simulink model "SAS"  (R2018a)
settings: Solver=VariableStepAuto  StartTime=0.0  StopTime=S.simtime  RelTol=1e-3
undefined symbols (not defined in the file): S
libraries: peGeneralControl x1
settings Model: Creator=Can Bekar  LastModifiedBy=Can Bekar
settings DataIOCC: ExternalInput=S.usignal  InitialState=xu  LoadExternalInput=on  SignalLogging=off  DSMLogging=off

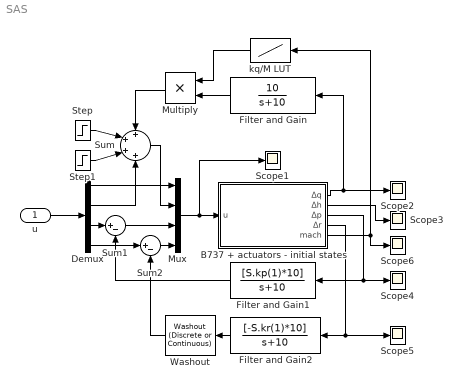
== system SAS ==
  u : Inport
  B737 + actuators - initial states : Subsystem
  Demux : Demux
  Filter and Gain : TransferFcn  Numerator=[10]  Denominator=[1 10]
  Filter and Gain1 : TransferFcn  Numerator=[S.kp(1)*10]  Denominator=[1 10]
  Filter and Gain2 : TransferFcn  Numerator=[-S.kr(1)*10]  Denominator=[1 10]
  Multiply : Product
  Mux : Mux
  Scope{1..6} (6 alike) : Scope
  Step : Step  Time=2  Before=deg2rad(1)  After=deg2rad(-1)  SampleTime=0
  Step1 : Step  After=deg2rad(1)  SampleTime=0
  Sum : Sum  Inputs=++++
  Sum1 : Sum  Inputs=|+-
  Sum2 : Sum  Inputs=|+-
  Washout : peGeneralControl/Washout (Discrete or Continuous)  T=1  Ts=-1
  kq/M LUT : Lookup_n-D  NumberOfTableDimensions=1  BreakpointsForDimension1=[0.2570 0.2590 0.2620 0.2640 0.2660 0.3510 0.3570 0.4200 0.4360 0.4520 0.4690 0.5440 0.5650 0.5870 0.6100 0.6340 0.6590 0.6850 0.7130 0.7270 0.7570 0.7800 0.7801 0.7802 0.7803 0.7804]  Table=S.kqLUT(:,2)  InternalRulePriority=Speed  RndMeth=Simplest  InputSameDT=on
  wires:
  Demux/1 -> Mux/1
  Sum/1 -> Mux/2
  Demux/2 -> Sum/4
  Mux/1 -> Scope1/1, B737 + actuators - initial states/1(u)
  u/1 -> Demux/1
  Step1/1 -> Sum/3
  Step/1 -> Sum/2
  Sum1/1 -> Mux/3
  Demux/3 -> Sum1/1
  Sum2/1 -> Mux/4
  Demux/4 -> Sum2/1
  Filter and Gain1/1 -> Sum1/2
  Filter and Gain2/1 -> Washout/1
  Washout/1 -> Sum2/2
  B737 + actuators - initial states/4(Δr) -> Scope5/1, Filter and Gain2/1
  B737 + actuators - initial states/1(Δq) -> Scope2/1, Filter and Gain/1
  B737 + actuators - initial states/3(Δp) -> Filter and Gain1/1, Scope4/1
  B737 + actuators - initial states/2(Δh) -> Scope3/1
  Filter and Gain/1 -> Multiply/2
  Multiply/1 -> Sum/1
  kq/M LUT/1 -> Multiply/1
  B737 + actuators - initial states/5(mach) -> Scope6/1, kq/M LUT/1

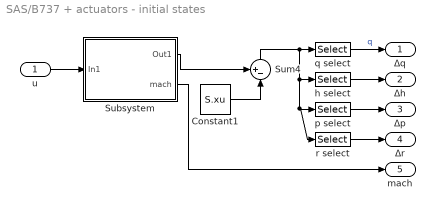
== system SAS/B737 + actuators - initial states ==
  u : Inport
  Constant1 : Constant  Value=S.xu
  Subsystem : Subsystem
  Sum4 : Sum  Inputs=+-|
  h select : Selector  InputPortWidth=12  IndexOptions=Index vector (dialog)  Indices=[12]  OutputSizes=1
  p select : Selector  InputPortWidth=12  IndexOptions=Index vector (dialog)  Indices=[7]  OutputSizes=1
  q select : Selector  InputPortWidth=12  IndexOptions=Index vector (dialog)  Indices=[8]  OutputSizes=1
  r select : Selector  InputPortWidth=12  IndexOptions=Index vector (dialog)  Indices=[9]  OutputSizes=1
  Δq : Outport
  Δh : Outport  Port=2
  Δp : Outport  Port=3
  Δr : Outport  Port=4
  mach : Outport  Port=5
  wires:
  q select/1 -> Δq/1  "q"
  r select/1 -> Δr/1
  Sum4/1 -> r select/1, p select/1, h select/1, q select/1
  Subsystem/1(Out1) -> Sum4/1
  u/1 -> Subsystem/1(In1)
  Constant1/1 -> Sum4/2
  h select/1 -> Δh/1
  p select/1 -> Δp/1
  Subsystem/2(mach) -> mach/1

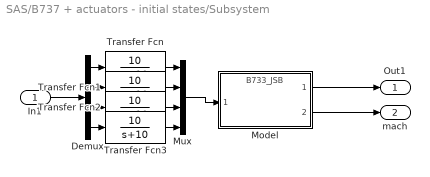
== system SAS/B737 + actuators - initial states/Subsystem ==
  In1 : Inport
  Demux : Demux
  Model : ModelReference  ModelNameDialog=B733_JSB  SimulationMode=Normal  ModelReferenceVersion=1.185
  Mux : Mux
  Transfer Fcn{,1..3} (4 alike) : TransferFcn  Numerator=[10]  Denominator=[1 10]
  Out1 : Outport
  mach : Outport  Port=2
  wires:
  In1/1 -> Demux/1
  Model/1 -> Out1/1
  Mux/1 -> Model/1
  Transfer Fcn/1 -> Mux/1
  Demux/1 -> Transfer Fcn/1
  Demux/2 -> Transfer Fcn1/1
  Transfer Fcn1/1 -> Mux/2
  Demux/3 -> Transfer Fcn2/1
  Transfer Fcn2/1 -> Mux/3
  Demux/4 -> Transfer Fcn3/1
  Transfer Fcn3/1 -> Mux/4
  Model/2 -> mach/1
